simulink library "anchorTetherCtrl_cl"  (R2018b)
settings: Solver=VariableStepAuto  StartTime=0.0  StopTime=10.0  RelTol=1e-3
undefined symbols (not defined in the file or in its folder): initializeBussesFromBlock
libraries: filteredPIDController_ul x3
settings Model: Creator=Erin B  LastModifiedBy=mcobb

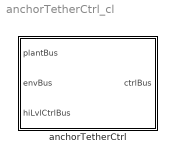
== system anchorTetherCtrl_cl ==
  anchorTetherCtrl : Subsystem  LoadFcn=initializeBussesFromBlock(gcb)  InitFcn=initializeBussesFromBlock(gcb)  StartFcn=initializeBussesFromBlock(gcb)  mask{ctrl=0}
      mask prompts: ctrl "Controller Object"

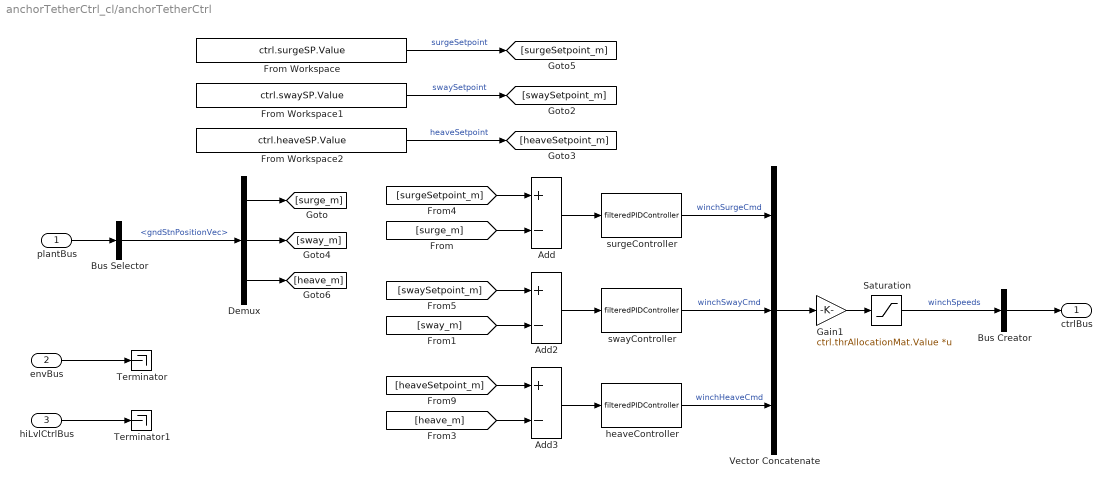
== system anchorTetherCtrl_cl/anchorTetherCtrl ==
  plantBus : Inport  OutDataTypeStr=Bus: plantBus
  envBus : Inport  Port=2  OutDataTypeStr=Bus: envBus
  hiLvlCtrlBus : Inport  Port=3  OutDataTypeStr=Bus: hiLvlCtrlBus
  Add : Sum  Inputs=+-
  Add2 : Sum  Inputs=+-
  Add3 : Sum  Inputs=+-
  Bus Creator : BusCreator  Inputs=1  OutDataTypeStr=Bus: gndStnCtrlBus
  Bus Selector : BusSelector  OutputSignals=gndStnPositionVec
  Demux : Demux  Outputs=3
  From Workspace : FromWorkspace  VariableName=ctrl.surgeSP.Value  SampleTime=0
  From Workspace1 : FromWorkspace  VariableName=ctrl.swaySP.Value  SampleTime=0
  From Workspace2 : FromWorkspace  VariableName=ctrl.heaveSP.Value  SampleTime=0
  Gain1 : Gain  Gain=ctrl.thrAllocationMat.Value  Multiplication=Matrix(K*u)
  Saturation : Saturate  UpperLimit=ctrl.outputSat.upperLimit.Value  LowerLimit=ctrl.outputSat.lowerLimit.Value
  Terminator : Terminator
  Terminator1 : Terminator
  Vector Concatenate : Concatenate  NumInputs=3
  heaveController : filteredPIDController_ul/filteredPIDController  kp=ctrl.heave.kp.Value  ki=ctrl.heave.ki.Value  kd=ctrl.heave.kd.Value  Value=ctrl.heave.tau.Value
  surgeController : filteredPIDController_ul/filteredPIDController  kp=ctrl.surge.kp.Value  ki=ctrl.surge.ki.Value  kd=ctrl.surge.kd.Value  Value=ctrl.surge.tau.Value
  swayController : filteredPIDController_ul/filteredPIDController  kp=ctrl.sway.kp.Value  ki=ctrl.sway.ki.Value  kd=ctrl.sway.kd.Value  Value=ctrl.sway.tau.Value
  ctrlBus : Outport  OutDataTypeStr=Bus: gndStnCtrlBus
  wires:
  Add3/1 -> heaveController/1
  Add2/1 -> swayController/1
  [swaySetpoint_m] -> Add2/1
  From Workspace/1 -> [surgeSetpoint_m]  "surgeSetpoint"
  [heaveSetpoint_m] -> Add3/1
  Gain1/1 -> Saturation/1
  surgeController/1 -> Vector Concatenate/1  "winchSurgeCmd"
  Add/1 -> surgeController/1
  [sway_m] -> Add2/2
  [heave_m] -> Add3/2
  heaveController/1 -> Vector Concatenate/3  "winchHeaveCmd"
  swayController/1 -> Vector Concatenate/2  "winchSwayCmd"
  [surgeSetpoint_m] -> Add/1
  Vector Concatenate/1 -> Gain1/1
  From Workspace1/1 -> [swaySetpoint_m]  "swaySetpoint"
  From Workspace2/1 -> [heaveSetpoint_m]  "heaveSetpoint"
  Demux/1 -> [surge_m]
  Demux/3 -> [heave_m]
  Demux/2 -> [sway_m]
  Saturation/1 -> Bus Creator/1  "winchSpeeds"
  [surge_m] -> Add/2
  plantBus/1 -> Bus Selector/1
  Bus Selector/1 -> Demux/1  "<gndStnPositionVec>"
  envBus/1 -> Terminator/1
  Bus Creator/1 -> ctrlBus/1
  hiLvlCtrlBus/1 -> Terminator1/1
